simulink model "LinearObserver"  (R2019b)
settings: Solver=FixedStepAuto  StartTime=0.0  StopTime=10.0  FixedStep=0.01  RelTol=1e-3
undefined symbols (not defined in the file): A, Aobs, B, Bobs, C, Cobs
settings Model: Creator=김태욱  LastModifiedBy=김태욱

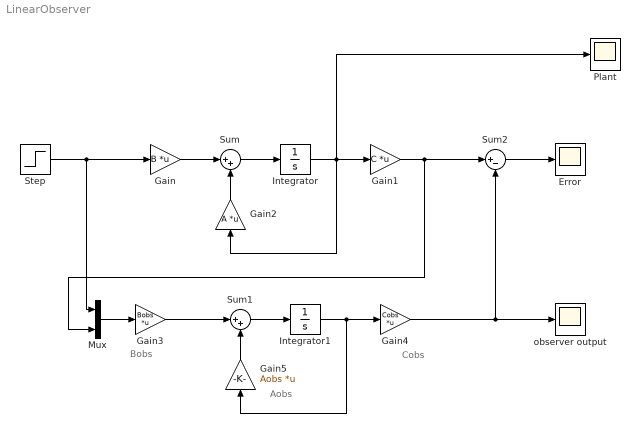
== system LinearObserver ==
  note: Cobs
  note: Aobs
  note: Bobs
  Error : Scope
  Gain : Gain  Gain=B  Multiplication=Matrix(K*u)
  Gain1 : Gain  Gain=C  Multiplication=Matrix(K*u)
  Gain2 : Gain  Gain=A  Multiplication=Matrix(K*u)
  Gain3 : Gain  Gain=Bobs  Multiplication=Matrix(K*u)
  Gain4 : Gain  Gain=Cobs  Multiplication=Matrix(K*u)
  Gain5 : Gain  Gain=Aobs  Multiplication=Matrix(K*u)
  Integrator : Integrator
  Integrator1 : Integrator  InitialCondition=[1;-1]
  Mux : Mux  Inputs=2
  Plant : Scope
  Step : Step  SampleTime=0
  Sum : Sum  Inputs=|++
  Sum1 : Sum  Inputs=|++
  Sum2 : Sum  Inputs=|+-
  observer output : Scope
  wires:
  Integrator/1 -> Plant/1, Gain2/1, Gain1/1
  Gain/1 -> Sum/1
  Sum/1 -> Integrator/1
  Gain2/1 -> Sum/2
  Gain5/1 -> Sum1/2
  Sum1/1 -> Integrator1/1
  Gain3/1 -> Sum1/1
  Integrator1/1 -> Gain4/1, Gain5/1
  Mux/1 -> Gain3/1
  Step/1 -> Gain/1, Mux/1
  Gain1/1 -> Sum2/1, Mux/2
  Gain4/1 -> observer output/1, Sum2/2
  Sum2/1 -> Error/1
